simulink library "csc_fps_feature_sensor_prep_lib"  (R2014b)
settings: Solver=ode45  SolverMode=SingleTasking  StartTime=0.0  StopTime=10.0  RelTol=1e-3
values from neighbouring files (symbols this model uses):
  fsp_camera_alt_cutoff = 5    [csc_snp_sensor_prep_init.m]
  snp_fsp_zero_index = [ 0 0 ]    [csc_snp_sensor_prep_init.m]
undefined symbols (not defined in the file or in its folder): P, x
libraries: simulink x1
settings Model: ExtModeAutoUpdateStatusClock=off  Creator=Administrator  LastModifiedBy=mstewart

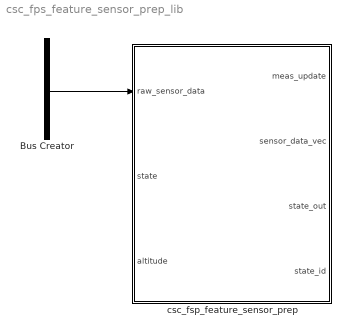
== system csc_fps_feature_sensor_prep_lib ==
  Bus Creator : BusCreator
  csc_fsp_feature_sensor_prep : Subsystem
  wires:
  ? -> Bus Creator/2  "accel"
  ? -> Bus Creator/3  "rate"
  ? -> Bus Creator/1  "x"
  ? -> Bus Creator/4  "q"
  Bus Creator/1 -> csc_fsp_feature_sensor_prep/1(raw_sensor_data)

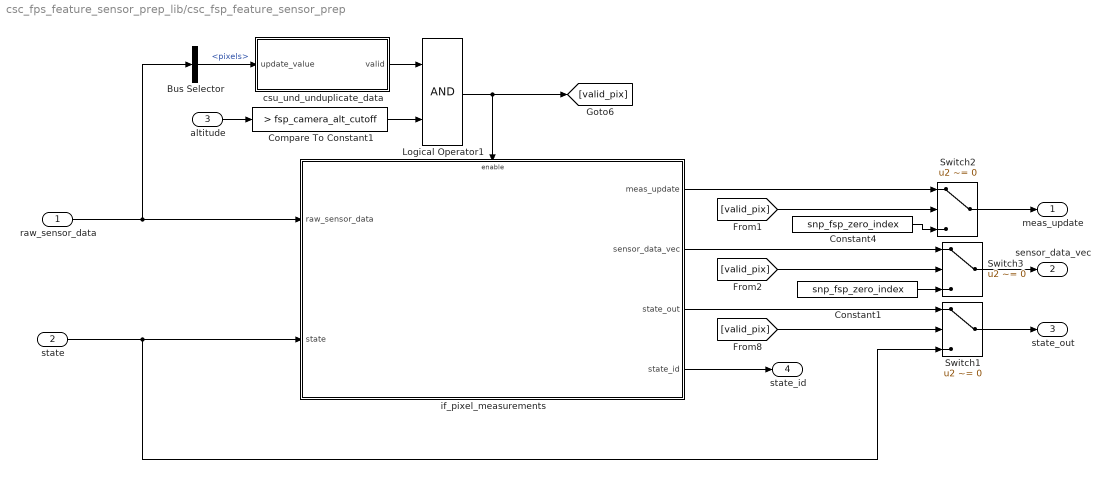
== system csc_fps_feature_sensor_prep_lib/csc_fsp_feature_sensor_prep ==
  raw_sensor_data : Inport
  state : Inport  Port=2
  altitude : Inport  Port=3
  Bus Selector : BusSelector  OutputSignals=pixels
  Compare To Constant1 : simulink/Logic and Bit Operations/Compare To Constant  relop=>  const=fsp_camera_alt_cutoff  OutDataTypeStr=uint8
  Constant1 : Constant  Value=snp_fsp_zero_index
  Constant4 : Constant  Value=snp_fsp_zero_index
  Logical Operator1 : Logic  AllPortsSameDT=off  OutDataTypeStr=boolean
  Switch1 : Switch  Criteria=u2 ~= 0
  Switch2 : Switch  Criteria=u2 ~= 0
  Switch3 : Switch  Criteria=u2 ~= 0
  csu_und_unduplicate_data : Subsystem  mask{initial_compare=0}
      mask prompts: initial_compare "initial comparison value"
      mask Display:
      | port_label('input',1,'update');
      | port_label('output',1','valid');
  if_pixel_measurements : Subsystem  TreatAsAtomicUnit=on
  meas_update : Outport
  sensor_data_vec : Outport  Port=2
  state_out : Outport  Port=3
  state_id : Outport  Port=4
  wires:
  raw_sensor_data/1 -> Bus Selector/1, if_pixel_measurements/1(raw_sensor_data)
  state/1 -> if_pixel_measurements/2(state), Switch1/3
  Bus Selector/1 -> csu_und_unduplicate_data/1(update_value)  "<pixels>"
  if_pixel_measurements/3(state_out) -> Switch1/1
  [valid_pix] -> Switch1/2
  Switch1/1 -> state_out/1
  [valid_pix] -> Switch2/2
  if_pixel_measurements/1(meas_update) -> Switch2/1
  Switch2/1 -> meas_update/1
  [valid_pix] -> Switch3/2
  if_pixel_measurements/2(sensor_data_vec) -> Switch3/1
  Switch3/1 -> sensor_data_vec/1
  Constant4/1 -> Switch2/3
  Constant1/1 -> Switch3/3
  if_pixel_measurements/4(state_id) -> state_id/1
  altitude/1 -> Compare To Constant1/1
  Compare To Constant1/1 -> Logical Operator1/2
  csu_und_unduplicate_data/1(valid) -> Logical Operator1/1
  Logical Operator1/1 -> [valid_pix], if_pixel_measurements/Enable

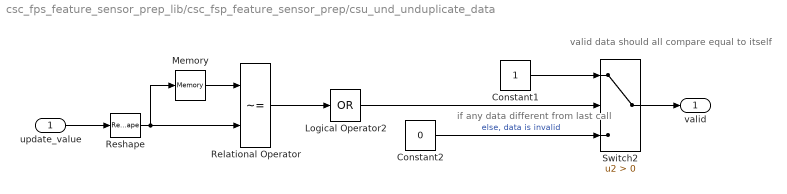
== system csc_fps_feature_sensor_prep_lib/csc_fsp_feature_sensor_prep/csu_und_unduplicate_data ==
  note: valid data should all compare equal to itself
  note: if any data different from last call
  update_value : Inport
  Constant1 : Constant
  Constant2 : Constant  Value=0
  Logical Operator2 : Logic  Operator=OR  Inputs=1  AllPortsSameDT=off  OutDataTypeStr=boolean
  Memory : Memory  X0=initial_compare  InheritSampleTime=on
  Relational Operator : RelationalOperator  Operator=~=  OutDataTypeStr=boolean
  Reshape : Reshape  OutputDimensionality=Customize  OutputDimensions=[30]
  Switch2 : Switch  Criteria=u2 > Threshold
  valid : Outport  InitialOutput=1
  wires:
  Logical Operator2/1 -> Switch2/2
  Memory/1 -> Relational Operator/1
  Constant2/1 -> Switch2/3  "else, data is invalid"
  Relational Operator/1 -> Logical Operator2/1
  update_value/1 -> Reshape/1
  Constant1/1 -> Switch2/1
  Switch2/1 -> valid/1
  Reshape/1 -> Memory/1, Relational Operator/2

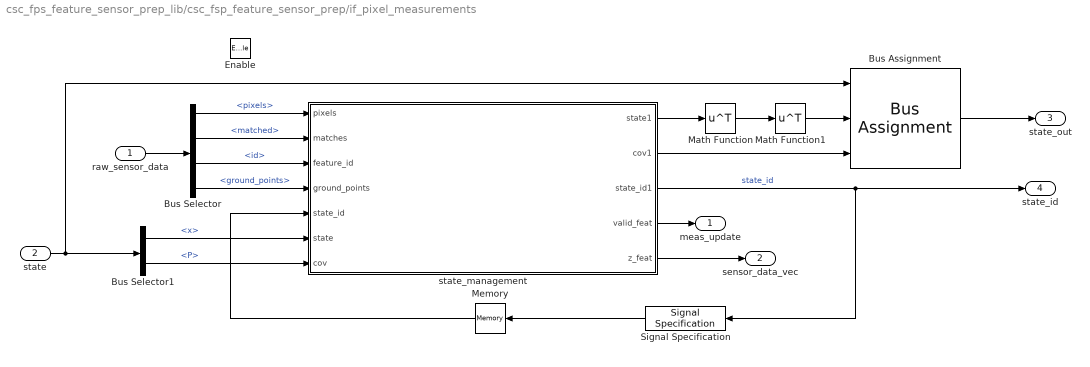
== system csc_fps_feature_sensor_prep_lib/csc_fsp_feature_sensor_prep/if_pixel_measurements ==
  raw_sensor_data : Inport
  state : Inport  Port=2
  Enable : EnablePort
  Bus Assignment : BusAssignment  AssignedSignals=x,P
  Bus Selector : BusSelector  OutputSignals=pixels,matched,id,ground_points
  Bus Selector1 : BusSelector  OutputSignals=x,P
  Math Function : Math  Operator=transpose  SaturateOnIntegerOverflow=on
  Math Function1 : Math  Operator=transpose  SaturateOnIntegerOverflow=on
  Memory : Memory  X0=zeros(24,1)  InheritSampleTime=on
  Signal Specification : SignalSpecification  OutDataTypeStr=double
  state_management : MATLAB Function  TreatAsAtomicUnit=on
  meas_update : Outport
  sensor_data_vec : Outport  Port=2
  state_out : Outport  Port=3
  state_id : Outport  Port=4
  wires:
  raw_sensor_data/1 -> Bus Selector/1
  state/1 -> Bus Assignment/1, Bus Selector1/1
  Bus Selector/1 -> state_management/1(pixels)  "<pixels>"
  Bus Selector/2 -> state_management/2(matches)  "<matched>"
  Bus Selector/3 -> state_management/3(feature_id)  "<id>"
  Bus Selector/4 -> state_management/4(ground_points)  "<ground_points>"
  state_management/4(valid_feat) -> meas_update/1
  state_management/5(z_feat) -> sensor_data_vec/1
  state_management/1(state1) -> Math Function/1
  state_management/3(state_id1) -> Signal Specification/1, state_id/1  "state_id"
  Memory/1 -> state_management/5(state_id)
  Math Function/1 -> Math Function1/1
  Math Function1/1 -> Bus Assignment/2
  Bus Selector1/1 -> state_management/6(state)  "<x>"
  Bus Selector1/2 -> state_management/7(cov)  "<P>"
  state_management/2(cov1) -> Bus Assignment/3
  Bus Assignment/1 -> state_out/1
  Signal Specification/1 -> Memory/1

== matlab function csc_fps_feature_sensor_prep_lib/csc_fsp_feature_sensor_prep/if_pixel_measurements/state_management ==
  data: pixels input; state1 output; cov1 output; matches input; feature_id input; ground_points input; state_id input; state input; state_id1 output; valid_feat output; z_feat output; cov input
function [state1,cov1, state_id1,valid_feat,z_feat] = state_management(pixels, matches, feature_id, ground_points, state_id, state, cov)
%#codegen

state1 = state;
state_id1 = state_id;
cov1 = cov;

n_feat = 3;

z_feat = zeros(n_feat*2,1);
valid_feat = zeros(n_feat*2,1);
feat_meas_id = zeros(n_feat*2,1);

% Look for current state features in measurements
current_feature_ids = state_id([16 19 22])';


% if the state has no features initialized
if all(current_feature_ids == 0)
    
    for ii = 1 : n_feat
        
        % take the first three features
        z_feat(2*(ii-1)+[1 2]) = pixels(10+ii,:)';
        valid_feat(2*(ii-1)+[1 2]) = 1;
        feat_meas_id(2*(ii-1)+[1 2]) = feature_id(10+ii);
        
        % add the ground points to the state vector
        state1(15 + 3*(ii-1)+[1 2 3]) = ground_points(10+ii,:)';
        state_id1(15 + 3*(ii-1)+[1 2 3]) = feature_id(10+ii);
        
    end
    
else
    % Capture which points were successfully matched
    points_matched = feature_id .* double(matches > 0);
    
    for ii = 1 : n_feat

        %feat_row_1 = find(points_matched == current_feature_ids(ii), 1);
        feat_row_1 = 0;
        if any(points_matched == current_feature_ids(ii));
           for pp = 1 : length(points_matched);
               if points_matched(pp) == current_feature_ids(ii);
                   feat_row_1 = pp;
                   break;
               end
           end
        end
        
        if feat_row_1 ~= 0
            % the current state feature has been measured again: update it
            z_feat(2*(ii-1)+[1 2]) = pixels(feat_row_1,:)';
            valid_feat(2*(ii-1)+[1 2]) = 1;
            feat_meas_id(2*(ii-1)+[1 2]) = current_feature_ids(ii);
            
        else
            
            % no valid measurement of that point
            % replace that point with a new one
            
            % find a good feature

            new_feature_row = -1;
            for kk = 1 : length(feature_id)

                if ~any(current_feature_ids == feature_id((kk))) && matches(kk) == 1
                    
                    new_feature_row = kk;
                    break
                    
                end
                
            end
            
            if new_feature_row > 0
                z_feat(2*(ii-1)+[1 2]) = pixels(new_feature_row,:)';
                valid_feat(2*(ii-1)+[1 2]) = 0;
                feat_meas_id(2*(ii-1)+[1 2]) = feature_id(new_feature_row);
                
                % add the ground points to the state vector
                state1(15 + 3*(ii-1)+[1 2 3]) = ground_points(new_feature_row,:)';
                state_id1(15 + 3*(ii-1)+[1 2 3]) = feature_id(new_feature_row);
                cov1(15 + 3*(ii-1)+[1 2 3], 15 + 3*(ii-1)+[1 2 3]) = 0.1*eye(3);
                
                current_feature_ids = state_id1([16 19 22])';
                
            else

                % invalid measurement
                z_feat(2*(ii-1)+[1 2]) = 0;
                valid_feat(2*(ii-1)+[1 2]) = 0;
                feat_meas_id(2*(ii-1)+[1 2]) = current_feature_ids(ii);
                
            end
            
        end
        
    end
end
